simulink subsystem "stack_model_subsystem"  (R2023a)
settings: Solver=VariableStepAuto  StartTime=0.0  StopTime=10.0  RelTol=1e-3
values from neighbouring files (symbols this model uses):
  constants =     [All_Properties.mat]
  coolant_initial_temperature = 313.15    [All_Properties.mat]    (also in cathode_subsystem_parameters.m = 293.15; thermal_subsystem_parameters.m = 293.15)
  env_p = 0.101325    [All_Properties.mat]    (also in Plant_Model_HT_Cooling_Parameters.m; anode_subsystem_parameters.m; environment_parameters.m; stack_model_harness_parameters.m)
  hydrogen =     [All_Properties.mat]
  oxygen =     [All_Properties.mat]
  stack_num_cells = 455    [All_Properties.mat]    (also in Plant_Model_HT_Cooling_Parameters.m = 400; cathode_subsystem_parameters.m; stack_model_parameters.m = 400; stack_subsystem_parameters.m)
undefined symbols (not defined in the file or in its folder): dewpoint_temperature_degC, h2_molar_concentration, inlet_flow_lpmin, inlet_pressure_barg, inlet_temperature_degC, stack, stoichiometry
libraries: fl_lib x28, nesl_utility x26
(part 2 of 2)

== matlab function stack_model_subsystem/evaluate_doe_model ==
  data: current input; anode_pressure_drop_mbar output; anode_temp_delta_degC output; cathode_pressure_drop_mbar output; cathode_temp_delta_degC output; cell_voltage_max_V output; cell_voltage_mean_V output; cell_voltage_min_V output; cell_voltage_std_dev_mV output; coolant_pressure_drop_mbar output; coolant_temp_delta_degC output; stack_voltage_V output; anode_supply input; stack_voltage_loss_V output; cathode_supply input; coolant_supply input
function [anode_pressure_drop_mbar, anode_temp_delta_degC, cathode_pressure_drop_mbar, ...
cathode_temp_delta_degC, cell_voltage_max_V, cell_voltage_mean_V, cell_voltage_min_V, ...
cell_voltage_std_dev_mV, coolant_pressure_drop_mbar, coolant_temp_delta_degC, ...
stack_voltage_V, stack_voltage_loss_V] = evaluate_doe_model(current, anode_supply, cathode_supply, coolant_supply)

% This function calls the .mex files created from PowerCell response
% surface interpolation of DoE data by providing the input arguments: 
% [current, anode_supply, cathode_supply, coolant_supply]. Note that the
% "model is only valid within the range of tested data." For more
% information, see: p10_doe_files\vendor_provision\Stack_Data_Model_Information.pdf

%% exclude .mex files from code generation

coder.extrinsic('get_anode_pressure_drop', 'get_anode_temp_delta', ...
    'get_cathode_pressure_drop', 'get_cathode_temp_delta', 'get_cell_voltage_max', ...
    'get_cell_voltage_mean', 'get_cell_voltage_min', 'get_cell_voltage_std_dev', ...
    'get_coolant_pressure_drop', 'get_coolant_temp_delta', 'get_stack_voltage', ...
    'get_stack_voltage_loss')

%% instantiate .mex file return variables as doubles

anode_pressure_drop_mbar = double(0);
anode_temp_delta_degC = double(0);
cathode_pressure_drop_mbar = double(0);
cathode_temp_delta_degC = double(0);
cell_voltage_max_V = double(0);
cell_voltage_mean_V = double(0);
cell_voltage_min_V = double(0);
cell_voltage_std_dev_mV = double(0);
coolant_pressure_drop_mbar = double(0);
coolant_temp_delta_degC = double(0);
stack_voltage_V = double(0);
stack_voltage_loss_V = double(0);

%% call .mex files created from PowerCell response surface interpolation of DoE data

anode_pressure_drop_mbar = get_anode_pressure_drop(current, ...
    anode_supply.h2_molar_concentration, anode_supply.stoichiometry, anode_supply.dewpoint_temperature_degC, anode_supply.inlet_temperature_degC, anode_supply.inlet_pressure_barg, ...
    cathode_supply.stoichiometry, cathode_supply.dewpoint_temperature_degC, cathode_supply.inlet_temperature_degC, cathode_supply.inlet_pressure_barg, ...
    coolant_supply.inlet_flow_lpmin, coolant_supply.inlet_temperature_degC);
anode_temp_delta_degC = get_anode_temp_delta(current, ...
    anode_supply.h2_molar_concentration, anode_supply.stoichiometry, anode_supply.dewpoint_temperature_degC, anode_supply.inlet_temperature_degC, anode_supply.inlet_pressure_barg, ...
    cathode_supply.stoichiometry, cathode_supply.dewpoint_temperature_degC, cathode_supply.inlet_temperature_degC, cathode_supply.inlet_pressure_barg, ...
    coolant_supply.inlet_flow_lpmin, coolant_supply.inlet_temperature_degC);
cathode_pressure_drop_mbar = get_cathode_pressure_drop(current, ...
    anode_supply.h2_molar_concentration, anode_supply.stoichiometry, anode_supply.dewpoint_temperature_degC, anode_supply.inlet_temperature_degC, anode_supply.inlet_pressure_barg, ...
    cathode_supply.stoichiometry, cathode_supply.dewpoint_temperature_degC, cathode_supply.inlet_temperature_degC, cathode_supply.inlet_pressure_barg, ...
    coolant_supply.inlet_flow_lpmin, coolant_supply.inlet_temperature_degC);
cathode_temp_delta_degC = get_cathode_temp_delta(current, ...
    anode_supply.h2_molar_concentration, anode_supply.stoichiometry, anode_supply.dewpoint_temperature_degC, anode_supply.inlet_temperature_degC, anode_supply.inlet_pressure_barg, ...
    cathode_supply.stoichiometry, cathode_supply.dewpoint_temperature_degC, cathode_supply.inlet_temperature_degC, cathode_supply.inlet_pressure_barg, ...
    coolant_supply.inlet_flow_lpmin, coolant_supply.inlet_temperature_degC);
cell_voltage_max_V = get_cell_voltage_max(current, ...
    anode_supply.h2_molar_concentration, anode_supply.stoichiometry, anode_supply.dewpoint_temperature_degC, anode_supply.inlet_temperature_degC, anode_supply.inlet_pressure_barg, ...
    cathode_supply.stoichiometry, cathode_supply.dewpoint_temperature_degC, cathode_supply.inlet_temperature_degC, cathode_supply.inlet_pressure_barg, ...
    coolant_supply.inlet_flow_lpmin, coolant_supply.inlet_temperature_degC);
cell_voltage_mean_V = get_cell_voltage_mean(current, ...
    anode_supply.h2_molar_concentration, anode_supply.stoichiometry, anode_supply.dewpoint_temperature_degC, anode_supply.inlet_temperature_degC, anode_supply.inlet_pressure_barg, ...
    cathode_supply.stoichiometry, cathode_supply.dewpoint_temperature_degC, cathode_supply.inlet_temperature_degC, cathode_supply.inlet_pressure_barg, ...
    coolant_supply.inlet_flow_lpmin, coolant_supply.inlet_temperature_degC);
cell_voltage_min_V = get_cell_voltage_min(current, ...
    anode_supply.h2_molar_concentration, anode_supply.stoichiometry, anode_supply.dewpoint_temperature_degC, anode_supply.inlet_temperature_degC, anode_supply.inlet_pressure_barg, ...
    cathode_supply.stoichiometry, cathode_supply.dewpoint_temperature_degC, cathode_supply.inlet_temperature_degC, cathode_supply.inlet_pressure_barg, ...
    coolant_supply.inlet_flow_lpmin, coolant_supply.inlet_temperature_degC);
cell_voltage_std_dev_mV = get_cell_voltage_std_dev(current, ...
    anode_supply.h2_molar_concentration, anode_supply.stoichiometry, anode_supply.dewpoint_temperature_degC, anode_supply.inlet_temperature_degC, anode_supply.inlet_pressure_barg, ...
    cathode_supply.stoichiometry, cathode_supply.dewpoint_temperature_degC, cathode_supply.inlet_temperature_degC, cathode_supply.inlet_pressure_barg, ...
    coolant_supply.inlet_flow_lpmin, coolant_supply.inlet_temperature_degC);
coolant_pressure_drop_mbar = get_coolant_pressure_drop(current, ...
    anode_supply.h2_molar_concentration, anode_supply.stoichiometry, anode_supply.dewpoint_temperature_degC, anode_supply.inlet_temperature_degC, anode_supply.inlet_pressure_barg, ...
    cathode_supply.stoichiometry, cathode_supply.dewpoint_temperature_degC, cathode_supply.inlet_temperature_degC, cathode_supply.inlet_pressure_barg, ...
    coolant_supply.inlet_flow_lpmin, coolant_supply.inlet_temperature_degC);
coolant_temp_delta_degC = get_coolant_temp_delta(current, ...
    anode_supply.h2_molar_concentration, anode_supply.stoichiometry, anode_supply.dewpoint_temperature_degC, anode_supply.inlet_temperature_degC, anode_supply.inlet_pressure_barg, ...
    cathode_supply.stoichiometry, cathode_supply.dewpoint_temperature_degC, cathode_supply.inlet_temperature_degC, cathode_supply.inlet_pressure_barg, ...
    coolant_supply.inlet_flow_lpmin, coolant_supply.inlet_temperature_degC);
stack_voltage_V = get_stack_voltage(current, ...
    anode_supply.h2_molar_concentration, anode_supply.stoichiometry, anode_supply.dewpoint_temperature_degC, anode_supply.inlet_temperature_degC, anode_supply.inlet_pressure_barg, ...
    cathode_supply.stoichiometry, cathode_supply.dewpoint_temperature_degC, cathode_supply.inlet_temperature_degC, cathode_supply.inlet_pressure_barg, ...
    coolant_supply.inlet_flow_lpmin, coolant_supply.inlet_temperature_degC);
stack_voltage_loss_V = get_stack_voltage_loss(current, ...
    anode_supply.h2_molar_concentration, anode_supply.stoichiometry, anode_supply.dewpoint_temperature_degC, anode_supply.inlet_temperature_degC, anode_supply.inlet_pressure_barg, ...
    cathode_supply.stoichiometry, cathode_supply.dewpoint_temperature_degC, cathode_supply.inlet_temperature_degC, cathode_supply.inlet_pressure_barg, ...
    coolant_supply.inlet_flow_lpmin, coolant_supply.inlet_temperature_degC);

== matlab function stack_model_subsystem/Stack Inner Calculations - Water production estimation/Saturation pressure of vapour water ==
  data: u input; y output
function y = fcn(u)

y =  0.61121 * exp((18.678 - (u / 234.5)) * (u / (257.14 + u)));;

== matlab function stack_model_subsystem/Stack Inner Calculations - Water production estimation/Saturation pressure of vapour water1 ==
  data: u input; y output
function y = fcn(u)

y =  0.61121 * exp((18.678 - (u / 234.5)) * (u / (257.14 + u)));;
